simulink model "rmaProjectSfunction"  (R2016b)
settings: Solver=VariableStepAuto  StartTime=0.0  StopTime=10.0  RelTol=1e-3
settings Model: Creator=Leo  LastModifiedBy=Leo

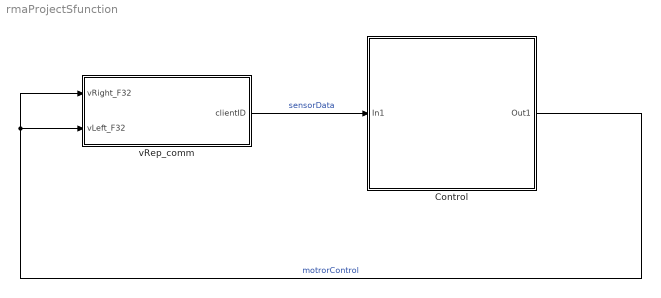
== system rmaProjectSfunction ==
  Control : Subsystem
      mask Display: image('LearnerGuideToSIMULINKA.png');
  vRep_comm : MATLAB Function  TreatAsAtomicUnit=on
  wires:
  vRep_comm/1(clientID) -> Control/1(In1)  "sensorData"
  Control/1(Out1) -> vRep_comm/2(vLeft_F32), vRep_comm/1(vRight_F32)  "motrorControl"

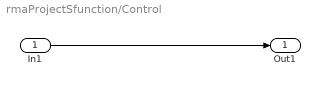
== system rmaProjectSfunction/Control ==
  In1 : Inport
  Out1 : Outport
  wires:
  In1/1 -> Out1/1

== matlab function rmaProjectSfunction/vRep_comm ==
  data: vRight_F32 input; clientID output; vLeft_F32 input
% Copyright 2017 Laercio Barbosa 
% leoabubauru@hotmail.com
% 
% -------------------------------------------------------------------
% THIS FILE IS DISTRIBUTED "AS IS", WITHOUT ANY EXPRESS OR IMPLIED
% WARRANTY. THE USER WILL USE IT AT HIS/HER OWN RISK. THE ORIGINAL
% AUTHOR AND COPPELIA ROBOTICS GMBH WILL NOT BE LIABLE FOR DATA LOSS,
% DAMAGES, LOSS OF PROFITS OR ANY OTHER KIND OF LOSS WHILE USING OR
% MISUSING THIS SOFTWARE.
% 
% You are free to use/modify/distribute this file for whatever purpose!
% -------------------------------------------------------------------
%

% Make sure to have the server side running in V-REP: 
% in a child script of a V-REP scene, add following command
% to be executed just once, at simulation start:
%
% simExtRemoteApiStart(19999)
%
% then start simulation, and run this matlab program.
%
% IMPORTANT: for each successful call to simxStart, there
% should be a corresponding call to simxFinish at the end!

function clientID  = vRep_comm(vRight_F32, vLeft_F32)
%RMAPROJECT V-REP remote control for a Pioneer robot
%   Controls Pioneer robot using Braitenberg algorithm in a V-REP simulation
persistent hasStarted;

    if (isempty(hasStarted) == true)
        hasStarted = false;
    end

    if (hasStarted == false)
        hasStarted = true;
        
        % Scene and pioneer motion variables
        sensorHandle = [0,0,0,0,0,0,0,0,0,0,0,0,0,0,0,0];
        state = [0,0,0,0,0,0,0,0,0,0,0,0,0,0,0,0];
        coord = struct('x', zeros(16), 'y', zeros(16), 'z', zeros(16));
        errVec = [1,1,1,1,1,1,1,1,1,1,1,1,1,1,1,1];

        disp('Program started');
        % vrep=remApi('remoteApi','extApi.h'); % using the header (requires a compiler)
        vrep = remApi('remoteApi'); % using the prototype file (remoteApiProto.m)
        vrep.simxFinish(-1); % just in case, close all opened connections
        clientID = vrep.simxStart('127.0.0.1',19999,true,true,5000,5);

        if (clientID > -1)
            disp('Connected to remote API server');
            % Now send some data to V-REP in a non-blocking fashion:
            vrep.simxAddStatusbarMessage(clientID,'Matlab remote client connected to V-REP!',vrep.simx_opmode_oneshot);

            % Motors initialization
            [erro, leftMotorHandle] = vrep.simxGetObjectHandle(clientID,'Pioneer_p3dx_leftMotor',vrep.simx_opmode_oneshot_wait);
            if (erro ~= 0)
                disp('Handle for left motor not found!');
            else
                disp('Connected to left motor!');
            end

            [erro, rightMotorHandle] = vrep.simxGetObjectHandle(clientID,'Pioneer_p3dx_rightMotor',vrep.simx_opmode_oneshot_wait);
            if (erro ~= vrep.simx_return_ok)
                disp('Handle for right motor not found!');
            else
                disp('Connected to right motor!');
            end

            % Sensors initialization (remoteApi)
            for i = 1:16
                [erro, sensorHandle(i)] = vrep.simxGetObjectHandle(clientID,['Pioneer_p3dx_ultrasonicSensor' num2str(i)],vrep.simx_opmode_oneshot_wait);
                if (erro ~= vrep.simx_return_ok)
                    disp(['Handle for sensor Pioneer_p3dx_ultrasonicSensor' num2str(i) ' not found!']);
                else
                    disp(['Connected to sensor Pioneer_p3dx_ultrasonicSensor' num2str(i) '!']);
                    % We start streaming data, but ignore function outputs as
                    % is the first call - see function help
                    [~, ~, ~, ~] = vrep.simxReadProximitySensor(clientID, sensorHandle(i),vrep.simx_opmode_streaming);
                end
            end
        else
            disp('Failed connecting to remote API server');
        end
    end        

    % Robot speed and deviation calculation. Runs until simulation has finished!
    if (vrep.simxGetConnectionId(clientID) ~= -1)
%         for i = 1:16
%             [errVec(i), state(i), coord(i), ~, ~] = vrep.simxReadProximitySensor(clientID, sensorHandle(i),vrep.simx_opmode_buffer);
%         end
        
        % Update motors speed
        vrep.simxSetJointTargetVelocity(clientID, leftMotorHandle, vLeft_F32, vrep.simx_opmode_streaming);
        vrep.simxSetJointTargetVelocity(clientID, rightMotorHandle, vRight_F32, vrep.simx_opmode_streaming);
    else

        % Before closing the connection to V-REP, make sure that the last command sent out had time to arrive. You can guarantee this with (for example):
        vrep.simxGetPingTime(clientID);

        % Now close the connection to V-REP:    
        vrep.simxFinish(clientID);
        
        % And stop simulation
        set_param(gcs, 'SimulationCommand', 'stop');

        disp('Program ended');
    end
end
